simulink model "lin121"  (R2021a)
settings: Solver=ode23tb  StartTime=0.0  StopTime=Tmdl  MaxStep=0.001  RelTol=1e-3
values from neighbouring files (symbols this model uses):
  lin =     [data.mat]
undefined symbols (not defined in the file or in its folder): k
settings Model: Creator=osini
settings DebuggingCC: UnconnectedInputMsg=none  UnconnectedOutputMsg=none  UnconnectedLineMsg=none
settings ModelReferenceCC: EnableRefExpFcnMdlSchedulingChecks=off
settings RTWCC: Description=Generic Real-Time Target  DLArmComputeVersion=20.02.1

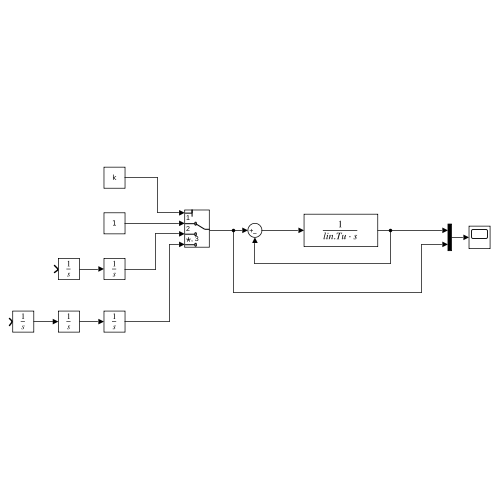
[thumbnail: Simulink's stored preview of the top-level diagram]
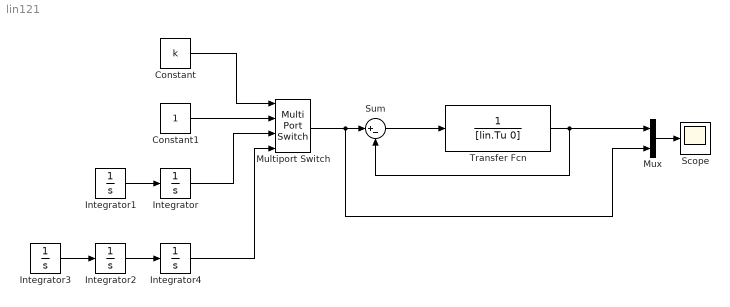
== system lin121 ==
  Constant : Constant  Value=k
  Constant1 : Constant
  Integrator : Integrator
  Integrator1 : Integrator  InitialCondition=1
  Integrator2 : Integrator
  Integrator3 : Integrator  InitialCondition=1
  Integrator4 : Integrator
  Multiport Switch : MultiPortSwitch
  Mux : Mux  Inputs=2
  Scope : Scope
  Sum : Sum  Inputs=|+-
  Transfer Fcn : TransferFcn  Denominator=[lin.Tu 0]
  wires:
  Sum/1 -> Transfer Fcn/1
  Transfer Fcn/1 -> Mux/1, Sum/2
  Constant/1 -> Multiport Switch/1
  Constant1/1 -> Multiport Switch/2
  Integrator/1 -> Multiport Switch/3
  Integrator2/1 -> Integrator4/1
  Integrator4/1 -> Multiport Switch/4
  Integrator3/1 -> Integrator2/1
  Integrator1/1 -> Integrator/1
  Mux/1 -> Scope/1
  Multiport Switch/1 -> Mux/2, Sum/1
